simulink model "lab14schema"  (R2023b)
settings: Solver=VariableStepAuto  StartTime=0.0  StopTime=5  RelTol=1e-3
values from neighbouring files (symbols this model uses):
  a = ws.A    [lab14.m]
  b = ws.B    [lab14.m]
  c = ws.C    [lab14.m]
  d = ws.D    [lab14.m]
undefined symbols (not defined in the file or in its folder): ae, be, ce, de
settings Model: Creator=user  LastModifiedBy=killer

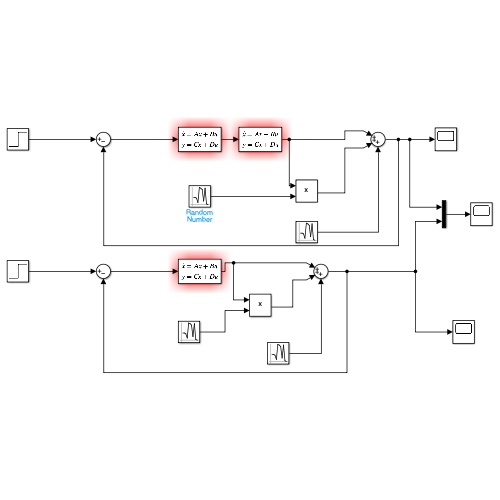
[thumbnail: Simulink's stored preview of the top-level diagram]
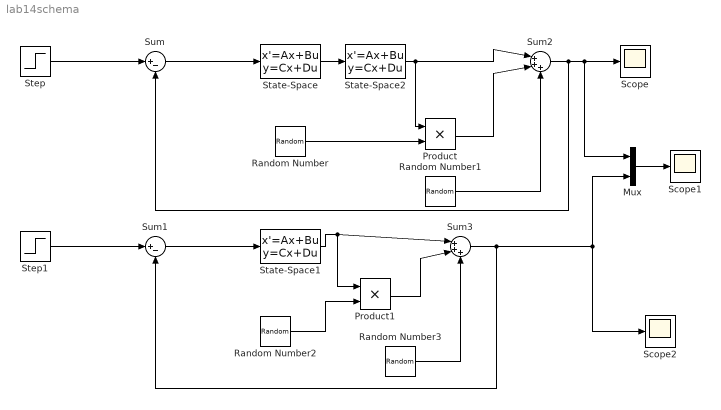
== system lab14schema ==
  Mux : Mux  Inputs=2
  Product : Product
  Product1 : Product
  Random Number{,1..3} (4 alike) : RandomNumber  Variance=0.05  SampleTime=0.1
  Scope : Scope
  Scope1 : Scope
  Scope2 : Scope
  State-Space : StateSpace  A=a  B=b  C=c  D=d  InitialCondition=0
  State-Space1 : StateSpace  A=ae  B=be  C=ce  D=de  InitialCondition=0
  State-Space2 : StateSpace  A=ae  B=be  C=ce  D=de  InitialCondition=0
  Step : Step  Time=0  SampleTime=0
  Step1 : Step  Time=0  SampleTime=0
  Sum : Sum  Inputs=|+-
  Sum1 : Sum  Inputs=|+-
  Sum2 : Sum  Inputs=|+++
  Sum3 : Sum  Inputs=|+++
  wires:
  Step/1 -> Sum/1
  Step1/1 -> Sum1/1
  Sum/1 -> State-Space/1
  State-Space/1 -> State-Space2/1
  State-Space2/1 -> Sum2/1, Product/1
  Product/1 -> Sum2/2
  Random Number/1 -> Product/2
  Random Number1/1 -> Sum2/3
  Sum2/1 -> Sum/2, Mux/1, Scope/1
  Mux/1 -> Scope1/1
  Sum1/1 -> State-Space1/1
  State-Space1/1 -> Product1/1, Sum3/1
  Random Number2/1 -> Product1/2
  Product1/1 -> Sum3/2
  Random Number3/1 -> Sum3/3
  Sum3/1 -> Sum1/2, Mux/2, Scope2/1
